simulink model "PNO_Module"  (R2024b)
settings: Solver=VariableStepAuto  StartTime=0.0  StopTime=10.0  RelTol=1e-3
undefined symbols (not defined in the file): stepUnit
settings Model: Creator=LiHaoh  LastModifiedBy=LiHaoh

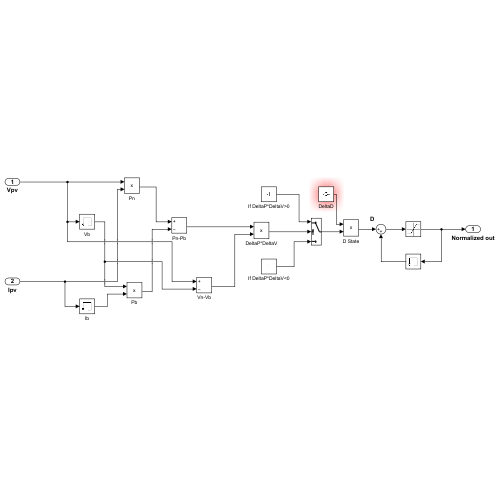
[thumbnail: Simulink's stored preview of the top-level diagram]
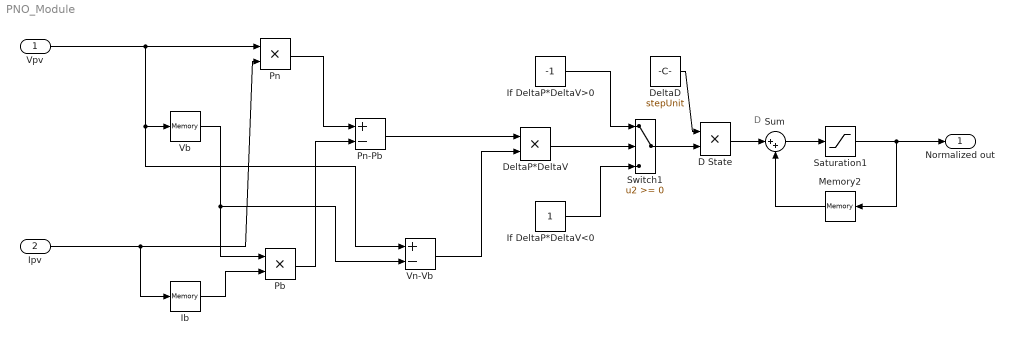
== system PNO_Module ==
  note: D
  Vpv : Inport
  Ipv : Inport  Port=2
  D State : Product  RndMeth=Zero
  DeltaD : Constant  Value=stepUnit
  DeltaP*DeltaV : Product  RndMeth=Zero
  Ib : Memory  InheritSampleTime=on  LinearizeAsDelay=on
  If DeltaP*DeltaV<0 : Constant
  If DeltaP*DeltaV>0 : Constant  Value=-1
  Memory2 : Memory  InheritSampleTime=on
  Pb : Product  RndMeth=Zero
  Pn : Product  RndMeth=Zero
  Pn-Pb : Sum  Inputs=+-
  Saturation1 : Saturate  UpperLimit=0.95  LowerLimit=0.1
  Sum : Sum  Inputs=|++
  Switch1 : Switch  SaturateOnIntegerOverflow=off  InputSameDT=off
  Vb : Memory  InheritSampleTime=on  LinearizeAsDelay=on
  Vn-Vb : Sum  Inputs=+-
  Normalized out : Outport
  wires:
  Pn/1 -> Pn-Pb/1
  Pn-Pb/1 -> DeltaP*DeltaV/1
  DeltaD/1 -> D State/1
  Vb/1 -> Vn-Vb/2, Pb/1
  Vpv/1 -> Vn-Vb/1, Vb/1, Pn/1
  Sum/1 -> Saturation1/1
  Ipv/1 -> Pn/2, Ib/1
  If DeltaP*DeltaV<0/1 -> Switch1/3
  Vn-Vb/1 -> DeltaP*DeltaV/2
  If DeltaP*DeltaV>0/1 -> Switch1/1
  Saturation1/1 -> Normalized out/1, Memory2/1
  DeltaP*DeltaV/1 -> Switch1/2
  Switch1/1 -> D State/2
  D State/1 -> Sum/1
  Memory2/1 -> Sum/2
  Pb/1 -> Pn-Pb/2
  Ib/1 -> Pb/2
